simulink library "neuromorphic_blocks"  (R2022a)
settings: Solver=VariableStepAuto  StartTime=0.0  StopTime=10.0  RelTol=1e-3
libraries: $bdroot x47, simulink x7
(part 2 of 3)

== system neuromorphic_blocks/Neural Blocks ==
  Modulatory Synapse : Subsystem  mask(Modulatory Synapse){base_val=0, gsyn_pos_source=Internal, gsyn_pos=0, gsyn_neg_source=Internal, gsyn_neg=0, timescale=0.004, rel_timescale=1000, input=Events, dsyn_pos=0, dsyn_neg=0, msyn_pos=1, msyn_neg=1}
      mask prompts: base_val "Value"; gsyn_pos_source "Source"; gsyn_pos "Value"; gsyn_neg_source "Source"; gsyn_neg "Value"; timescale "Value"; rel_timescale "Value"; dsyn_pos "Value"; dsyn_neg "Value"; msyn_pos "Value"; msyn_neg "Value"
      mask init: same as neuromorphic_blocks/Auxiliary Blocks/Event-Triggered Relay
      mask TypeOptions gsyn_pos_source: Internal | External
      mask Callback gsyn_pos_source:
      | mask  = Simulink.Mask.get(gcb);
      |     switch mask.getParameter('gsyn_pos_source').Value
      |         case 'Internal'
      |             mask.getParameter('gsyn_pos').Enabled = 'on';
      |         case 'External'
      |             mask.getParameter('gsyn_pos').Enabled = 'off';
      |     end
      mask TypeOptions gsyn_neg_source: Internal | External
      mask Callback gsyn_neg_source:
      | mask  = Simulink.Mask.get(gcb);
      |     switch mask.getParameter('gsyn_neg_source').Value
      |         case 'Internal'
      |             mask.getParameter('gsyn_neg').Enabled = 'on';
      |         case 'External'
      |             mask.getParameter('gsyn_neg').Enabled = 'off';
      |     end
      mask TypeOptions input: Events | Voltage
      mask Callback input:
      | mask = Simulink.Mask.get(gcb);
      |     switch mask.getParameter('input').Value
      |         case 'Events'
      |             mask.getParameter('dsyn_pos').Enabled = 'off';
      |             mask.getParameter('dsyn_pos').Visible = 'off';
      |             mask.getDialogControl('dsyn_pos_text').Enabled = 'off';
      |             mask.getDialogControl('dsyn_pos_text').Visible = 'off';
      |             mask.getParameter('dsyn_neg').Enabled = 'off';
      |             mask.getParameter('dsyn_neg').Visible = 'off';
      |             mask.getDialogControl('dsyn_neg_text').Enabled = 'off';
      |             mask.getDialogControl('dsyn_neg_text').Visible = 'off';
      |             mask.getParameter('msyn_pos').Enabled = 'off';
      |             mask.getParameter('msyn_pos').Visible = 'off';
      |             mask.getDialogControl('msyn_pos_text').Enabled = 'off';
      |             mask.getDialogControl('msyn_pos_text').Visible = 'off';
      |             mask.getParameter('msyn_neg').Enabled = 'off';
      |             mask.getParameter('msyn_neg').Visible = 'off';
      |             mask.getDialogControl('msyn_neg_text').Enabled = 'off';
      |             mask.getDialogControl('msyn_neg_text').Visible = 'off';
      |         case 'Voltage'
      |             mask.getParameter('dsyn_pos').Enabled = 'on';
      |             mask.getParameter('dsyn_pos').Visible = 'on';
      |             mask.getDialogControl('dsyn_pos_text').Enabled = 'on';
      |             mask.getDialogControl('dsyn_pos_text').Visible = 'on';
      |             mask.getParameter('dsyn_neg').Enabled = 'on';
      |             mask.getParameter('dsyn_neg').Visible = 'on';
      |             mask.getDialogControl('dsyn_neg_text').Enabled = 'on';
      |             mask.getDialogControl('dsyn_neg_text').Visible = 'on';
      |             mask.getParameter('msyn_pos').Enabled = 'on';
      |             mask.getParameter('msyn_pos').Visible = 'on';
      |             mask.getDialogControl('msyn_pos_text').Enabled = 'on';
      |             mask.getDialogControl('msyn_pos_text').Visible = 'on';
      |             mask.getParameter('msyn_neg').Enabled = 'on';
      |             mask.getParameter('msyn_neg').Visible = 'on';
      |             mask.getDialogControl('msyn_neg_text').Enabled = 'on';
      |             mask.getDialogControl('msyn_neg_text').Visible = 'on';
      |     end
      mask DialogControl base_val_text Prompt: Start Parameter
      mask DialogControl gsyn_pos_text Prompt: Positive Event Conductance
      mask DialogControl gsyn_neg_text Prompt: Negative Event Conductance
      mask DialogControl timescale_text Prompt: Timescale
      mask DialogControl rel_timescale_text Prompt: Relative Timescale
      mask DialogControl input_text Prompt: Input Type
      mask DialogControl dsyn_pos_text Prompt: Positive Event Bias
      mask DialogControl dsyn_neg_text Prompt: Negative Event Bias
      mask DialogControl msyn_pos_text Prompt: Positive Event Gain
      mask DialogControl msyn_neg_text Prompt: Negative Event Gain
      mask Display:
      | image('icons/modulatory.jpg');
      | 
      | port_label('output', 1, 'p');
      | 
      | simBlockH = get_param(gcb, 'Handle');
      | portH = find_system(simBlockH, 'LookUnderMasks', 'on', 'FollowLinks', 'on', 'SearchDepth', 1, 'BlockType', 'Inport');
      | portNames = cellstr(get_param(portH, 'Name'));
      | portNum = cellstr(get_param(portH, 'Port'));
      | for i = 1:length(portNames)
      |     if ~isempty(portNames{i})
      |         num = str2num(['uint8(' portNum{i} ')']);
      |         port_label('input', num, portNames{i});
      |     end
      | end
  Neuron : Subsystem  mask(Neuron){gfm_source=Internal, gfm=0, gsp_source=Internal, gsp=0, gsm_source=Internal, gsm=0, gup_source=Internal, gup=0, gum_source=Internal, gum=0, dfm=0, dsp=0, dsm=0, dup=0, dum=0, mfm=1, msp=1, msm=1, mup=1, mum=1, timescale=0.004, rel_membrane=0.1, rel_fast=0.1, rel_slow=4, rel_ultraslow=200, Iapp_base=0, V0=0, tresh=0, output=Events}
      mask prompts: gfm_source "Source"; gfm "Value"; gsp_source "Source"; gsp "Value"; gsm_source "Source"; gsm "Value"; gup_source "Source"; gup "Value"; gum_source "Source"; gum "Value"; dfm "Value"; dsp "Value"; dsm "Value"; dup "Value"; dum "Value"; mfm "Value"; msp "Value"; msm "Value"; mup "Value"; mum "Value"; timescale "Value"; rel_membrane "Value"; rel_fast "Value"; rel_slow "Value"; rel_ultraslow "Value"; Iapp_base "Value"; V0 "Value"; tresh "Value"
      mask help:
      | Block simulating a simplified neuron model (L. Ribar and R. Sepulchre 2019).
      | The conductances can either be set or given as external inputs for neuromodulation.
      mask init:
      | mask  = Simulink.Mask.get(gcb);
      |     
      |     suffix_list = {'fm','sp','sm','up','um'};
      |     
      |     for suffix_cell = suffix_list
      |         suffix = suffix_cell{1};
      |         %block = find_system(gcb, 'LookUnderMasks', 'on', ...
      |         %                        'FollowLinks', 'on', 'Name', ['g' suffix]);
      |         %if isempty(block) 
      |             % Something is very wrong, recreate block
      |         %    add_block('built-in/Constant', [gcb '/g' suffix])
      |         %    h = get_param([gcb '/I' suffix],'LineHandles');
      |         %    if h.Inport(2) > 0
      |         %        delete_line(h.Inport(2)); 
      |         %    end 
      |         %    add_line(gcb,['g' suffix '/1'],['I' suffix '/2']);
      |         %end
      |     
      |         type = get_param([gcb '/g' suffix],'BlockType');
      |         switch mask.getParameter(['g' suffix '_source']).Value
      |             case 'Internal'
      |                 switch type
      |                     case 'Inport'
      |                         replace_block([gcb '/g' suffix], 'Inport', 'Constant', 'noprompt');
      |                         set_param([gcb '/g' suffix],'Value',['g' suffix]);
      |                 end
      |                 if strcmp('0', mask.getParameter(['g' suffix ]).Value)
      |                     set_param([gcb '/I' suffix],'Commented','on')
      |                     set_param([gcb '/g' suffix],'Commented','on')
      |                     set_param([gcb '/I' suffix '_sub'],'Commented','on')
      |                 else
      |                     set_param([gcb '/I' suffix],'Commented','off')
      |                     set_param([gcb '/g' suffix],'Commented','off')
      |                     set_param([gcb '/I' suffix '_sub'],'Commented','off')
      |                 end
      |             case 'External'
      |                 switch type
      |                     case 'Constant'
      |                         replace_block([gcb '/g' suffix], 'Constant', 'Inport', 'noprompt');
      |                 end
      |                 set_param([gcb '/I' suffix],'Commented','off')
      |                 set_param([gcb '/g' suffix],'Commented','off')
      |                 set_param([gcb '/I' suffix '_sub'],'Commented','off')
      |         end
      |     end
      | 
      |     type_V = get_param([gcb '/V'],'BlockType');
      |     type_Ev = get_param([gcb '/Ev'],'BlockType');
      |     switch mask.getParameter('output').Value
      |         case 'Events'
      |             switch type_V
      |                 case 'Outport'
      |                     replace_block([gcb '/V'], 'Outport', 'Terminator', 'noprompt')
      |             end
      |             switch type_Ev
      |                 case 'Terminator'
      |                     replace_block([gcb '/Ev'], 'Terminator', 'Outport', 'noprompt')
      |             end
      |             set_param([gcb '/V_to_Ev'],'Commented','off')
      |         case 'Voltage'
      |             switch type_V
      |                 case 'Terminator'
      |                     replace_block([gcb '/V'], 'Terminator', 'Outport', 'noprompt')
      |             end
      |             switch type_Ev
      |                 case 'Outport'
      |                     replace_block([gcb '/Ev'], 'Outport', 'Terminator', 'noprompt')
      |             end
      |             set_param([gcb '/V_to_Ev'],'Commented','on')
      |         case 'Both'
      |             switch type_Ev
      |                 case 'Terminator'
      |                     switch type_V
      |                         case 'Outport'
      |                             replace_block([gcb '/V'], 'Outport', 'Terminator', 'noprompt')
      |                             type_V = 'Terminator';
      |                     end
      |                     replace_block([gcb '/Ev'], 'Terminator', 'Outport', 'noprompt')
      |             end
      |             switch type_V
      |                 case 'Terminator'
      |                     replace_block([gcb '/V'], 'Terminator', 'Outport', 'noprompt')
      |             end
      |             set_param([gcb '/V_to_Ev'],'Commented','off')
      |     end
      mask TypeOptions gfm_source: Internal | External
      mask Callback gfm_source:
      | source_name = 'gfm_source';
      |     tgt_name = 'gfm';
      |     mask  = Simulink.Mask.get(gcb);
      |     switch mask.getParameter(source_name).Value
      |         case 'Internal'
      |             mask.getParameter(tgt_name).Enabled = 'on';
      |         case 'External'
      |             mask.getParameter(tgt_name).Enabled = 'off';
      |     end
      mask TypeOptions gsp_source: Internal | External
      mask Callback gsp_source:
      | source_name = 'gsp_source';
      |     tgt_name = 'gsp';
      |     mask  = Simulink.Mask.get(gcb);
      |     switch mask.getParameter(source_name).Value
      |         case 'Internal'
      |             mask.getParameter(tgt_name).Enabled = 'on';
      |         case 'External'
      |             mask.getParameter(tgt_name).Enabled = 'off';
      |     end
      mask TypeOptions gsm_source: Internal | External
      mask Callback gsm_source:
      | source_name = 'gsm_source';
      |     tgt_name = 'gsm';
      |     mask  = Simulink.Mask.get(gcb);
      |     switch mask.getParameter(source_name).Value
      |         case 'Internal'
      |             mask.getParameter(tgt_name).Enabled = 'on';
      |         case 'External'
      |             mask.getParameter(tgt_name).Enabled = 'off';
      |     end
      mask TypeOptions gup_source: Internal | External
      mask Callback gup_source:
      | source_name = 'gup_source';
      |     tgt_name = 'gup';
      |     mask  = Simulink.Mask.get(gcb);
      |     switch mask.getParameter(source_name).Value
      |         case 'Internal'
      |             mask.getParameter(tgt_name).Enabled = 'on';
      |         case 'External'
      |             mask.getParameter(tgt_name).Enabled = 'off';
      |     end
      mask TypeOptions gum_source: Internal | External
      mask Callback gum_source:
      | source_name = 'gum_source';
      |     tgt_name = 'gum';
      |     mask  = Simulink.Mask.get(gcb);
      |     switch mask.getParameter(source_name).Value
      |         case 'Internal'
      |             mask.getParameter(tgt_name).Enabled = 'on';
      |         case 'External'
      |             mask.getParameter(tgt_name).Enabled = 'off';
      |     end
      mask TypeOptions output: Events | Voltage | Both
      mask Callback output:
      | source_name = 'output';
      |     tgt_name = 'tresh';
      |     mask  = Simulink.Mask.get(gcb);
      |     switch mask.getParameter(source_name).Value
      |         case 'Voltage'
      |             mask.getParameter(tgt_name).Enabled = 'off';
      |         otherwise
      |             mask.getParameter(tgt_name).Enabled = 'on';
      |     end
      mask DialogControl ConductancesContainer Prompt: Conductances
      mask DialogControl gfm_text Prompt: Fast Negative Conductance (gfm)
      mask DialogControl gsp_text Prompt: Slow Positive Conductance (gsp)
      mask DialogControl gsm_text Prompt: Slow Negative Conductance (gsm)
      mask DialogControl gup_text Prompt: Ultra-Slow Positive Conductance (gup)
      mask DialogControl gum_text Prompt: Ultra-Slow Negative Conductance (gum)
      mask DialogControl BiasesContainer Prompt: Biases
      mask DialogControl dfm_text Prompt: Fast Negative Bias (dfm)
      mask DialogControl dsp_text Prompt: Slow Positive Bias (dsp)
      mask DialogControl dsm_text Prompt: Slow Negative Bias (dsm)
      mask DialogControl dup_text Prompt: Ultra-Slow Positive Bias (gup)
      mask DialogControl dum_text Prompt: Ultra-Slow Negative Bias (gum)
      mask DialogControl SlopesContainer Prompt: Slopes
      mask DialogControl mfm_text Prompt: Fast Negative Slope (mfm)
      mask DialogControl msp_text Prompt: Slow Positive Slope (msp)
      mask DialogControl msm_text Prompt: Slow Negative Slope (msm)
      mask DialogControl mup_text Prompt: Ultra-Slow Positive Slope (mup)
      mask DialogControl mum_text Prompt: Ultra-Slow Negative Slope (mum)
      mask DialogControl TimescalesContainer Prompt: Timescales
      mask DialogControl timescale_text Prompt: Timescale
      mask DialogControl memb_text Prompt: Relative Membrane Timescale
      mask DialogControl fast_text Prompt: Relative Fast Timescale
      mask DialogControl slow_text Prompt: Relative Slow Timescale
      mask DialogControl ultraslow_text Prompt: Relative Ultra-Slow Timescale
      mask DialogControl OtherContainer Prompt: Other
      mask DialogControl Iapp_text Prompt: Base Applied Current
      mask DialogControl V0_text Prompt: Base Voltage
      mask DialogControl tresh_text Prompt: Event Threshold
      mask DialogControl output_text Prompt: Output
      mask Display:
      | pos = get_param(gcb, 'Position');
      | width = pos(3) - pos(1);
      | height = pos(4) - pos(2);
      | 
      | image('icons/neuron.jpg');
      | 
      | simBlockH = get_param(gcb, 'Handle');
      | 
      | 
      | portH = find_system(simBlockH, 'LookUnderMasks', 'on', 'FollowLinks', 'on', 'SearchDepth', 1, 'BlockType', 'Inport');
      | portNames = cellstr(get_param(portH, 'Name'));
      | portNum = cellstr(get_param(portH, 'Port'));
      | for i = 1:length(portNames)
      |     if ~isempty(portNames{i})
      |         num = str2num(['uint8(' portNum{i} ')']);
      |         port_label('input', num, portNames{i});
      |     end
      | end
      | 
      | portH = find_system(simBlockH, 'LookUnderMasks', 'on', 'FollowLinks', 'on', 'SearchDepth', 1, 'BlockType', 'Outport');
      | portNames = cellstr(get_param(portH, 'Name'));
      | portNum = cellstr(get_param(portH, 'Port'));
      | for i = 1:length(portNames)
      |     if ~isempty(portNames{i})
      |         num = str2num(['uint8(' portNum{i} ')']);
      |         port_label('output', num, portNames{i});
      |     end
      | end
  Synapse with Depression : Subsystem  mask(Synapse with Depression){gsyn_source=Internal, gsyn=0, dsyn=0, msyn=1, dsyn_dep=0, msyn_dep=1, timescale=0.004, rel_facilitation=0, rel_depression=100, input=Events, gsyn_in=0, dsyn_in=0, msyn_in=1}
      mask prompts: gsyn_source "Source"; gsyn "Value"; dsyn "Value"; msyn "Value"; dsyn_dep "Value"; msyn_dep "Value"; timescale "Value"; rel_facilitation "Value"; rel_depression "Value"; gsyn_in "Value"; dsyn_in "Value"; msyn_in "Value"
      mask help: Synapse that lets through the first spikes
      mask init:
      | mask  = Simulink.Mask.get(gcb);
      |     %block = find_system(gcb, 'LookUnderMasks', 'on', ...
      |     %                    'FollowLinks', 'on', 'Name', 'gsyn');
      |     %if isempty(block) 
      |         % Something is very wrong, recreate block
      |     %    add_block('built-in/Constant', [gcb '/gsyn'])
      |     %    h = get_param([gcb '/Sigmoid'],'LineHandles');
      |     %    if h.Inport(2) > 0
      |     %        delete_line(h.Inport(2)); 
      |     %    end 
      |     %    add_line(gcb,'gsyn/1','Sigmoid/2');
      |     %    h = get_param([gcb '/Out Depression Sigmoid'],'LineHandles');
      |     %    if h.Inport(2) > 0
      |     %        delete_line(h.Inport(2)); 
      |     %    end 
      |     %    add_line(gcb,'gsyn/1','Out Depression Sigmoid/2');
      |     %end
      | 
      |     switch mask.getParameter('input').Value
      |         case 'Events'
      |             set_param([gcb '/VSNK' ],'LabelModeActiveChoice', 'Events');
      |             set_param([gcb '/VSRC' ],'LabelModeActiveChoice', 'Events');
      |             %mask.getPortConstraint('in_main_type').Rule.DataType = {'boolean'};
      |             try
      |                 set_param([gcb '/V'], 'Name', 'Ev');
      |             catch E
      |             end
      |         case 'Voltage'
      |             set_param([gcb '/VSNK' ],'LabelModeActiveChoice', 'Voltage');
      |             set_param([gcb '/VSRC' ],'LabelModeActiveChoice', 'Voltage');
      |             %mask.getPortConstraint('in_main_type').Rule.DataType = {'double'; 'single'; 'int8'; 'uint8'; 'int16'; 'uint16'; 'int32'; 'uint32'};
      |             try
      |                 set_param([gcb '/Ev'], 'Name', 'V');
      |             catch E
      |             end
      |     end
      | 
      |     switch mask.getParameter('gsyn_source').Value
      |         case 'Internal'
      |             replace_block([gcb '/gsyn'], 'Inport', 'Constant', 'noprompt');
      |             set_param([gcb '/gsyn'],'Value','gsyn');
      |         case 'External'
      |             replace_block([gcb '/gsyn'], 'Constant', 'Inport', 'noprompt');
      |     end
      mask TypeOptions gsyn_source: Internal | External
      mask Callback gsyn_source:
      | mask  = Simulink.Mask.get(gcb);
      |     switch mask.getParameter('gsyn_source').Value
      |         case 'Internal'
      |             mask.getParameter('gsyn').Enabled = 'on';
      |         case 'External'
      |             mask.getParameter('gsyn').Enabled = 'off';
      |     end
      mask TypeOptions input: Events | Voltage
      mask Callback input:
      | mask = Simulink.Mask.get(gcb);
      |     switch mask.getParameter('input').Value
      |         case 'Events'
      |             mask.getParameter('gsyn_in').Enabled = 'off';
      |             mask.getParameter('gsyn_in').Visible = 'off';
      |             mask.getDialogControl('gsyn_in_text').Enabled = 'off';
      |             mask.getDialogControl('gsyn_in_text').Visible = 'off';
      |             mask.getParameter('dsyn_in').Enabled = 'off';
      |             mask.getParameter('dsyn_in').Visible = 'off';
      |             mask.getDialogControl('dsyn_in_text').Enabled = 'off';
      |             mask.getDialogControl('dsyn_in_text').Visible = 'off';
      |             mask.getParameter('msyn_in').Enabled = 'off';
      |             mask.getParameter('msyn_in').Visible = 'off';
      |             mask.getDialogControl('msyn_in_text').Enabled = 'off';
      |             mask.getDialogControl('msyn_in_text').Visible = 'off';
      |         case 'Voltage'
      |             mask.getParameter('gsyn_in').Enabled = 'on';
      |             mask.getParameter('gsyn_in').Visible = 'on';
      |             mask.getDialogControl('gsyn_in_text').Enabled = 'on';
      |             mask.getDialogControl('gsyn_in_text').Visible = 'on';
      |             mask.getParameter('dsyn_in').Enabled = 'on';
      |             mask.getParameter('dsyn_in').Visible = 'on';
      |             mask.getDialogControl('dsyn_in_text').Enabled = 'on';
      |             mask.getDialogControl('dsyn_in_text').Visible = 'on';
      |             mask.getParameter('msyn_in').Enabled = 'on';
      |             mask.getParameter('msyn_in').Visible = 'on';
      |             mask.getDialogControl('msyn_in_text').Enabled = 'on';
      |             mask.getDialogControl('msyn_in_text').Visible = 'on';
      |     end
      mask DialogControl gsyn_text Prompt: Conductance (gsyn)
      mask DialogControl dsyn_text Prompt: Bias (dsyn)
      mask DialogControl msyn_text Prompt: Slope (msyn)
      mask DialogControl dsyn_dep_text Prompt: Depression Bias (dsyn_dep)
      mask DialogControl msyn_dep_text Prompt: Depression Slope (msyn_dep)
      mask DialogControl timescale_text Prompt: Timescale
      mask DialogControl rel_facilitation_text Prompt: Facilitation Timescale
      mask DialogControl rel_depression_text Prompt: Depression Timescale
      mask DialogControl input_text Prompt: Input Type
      mask DialogControl gsyn_in_text Prompt: Input Conductance (gsyn_in)
      mask DialogControl dsyn_in_text Prompt: Inout Bias (dsyn_in)
      mask DialogControl msyn_in_text Prompt: Input Slope (msyn_in)
      mask Display:
      | mask  = Simulink.Mask.get(gcb);
      | [gsyn, gsyn_converted] = str2num(mask.getParameter('gsyn').Value);
      | [msyn, msyn_converted] = str2num(mask.getParameter('msyn').Value);
      | 
      | if strcmp(mask.getParameter('gsyn_source').Value,'Internal') ...
      |    && gsyn_converted && msyn_converted && gsyn*msyn < 0
      |     image('icons/depressing_inhib_syn.jpg');
      | else
      |     image('icons/depressing_excit_syn.jpg');
      | end
      | 
      | port_label('output', 1, 'Isyn');
      | 
      | simBlockH = get_param(gcb, 'Handle');
      | portH = find_system(simBlockH, 'LookUnderMasks', 'on', 'FollowLinks', 'on', 'SearchDepth', 1, 'BlockType', 'Inport');
      | portNames = cellstr(get_param(portH, 'Name'));
      | portNum = cellstr(get_param(portH, 'Port'));
      | for i = 1:length(portNames)
      |     if ~isempty(portNames{i})
      |         num = str2num(['uint8(' portNum{i} ')']);
      |         port_label('input', num, portNames{i});
      |     end
      | end
  Synapse with Facilitation : Subsystem  mask(Synapse with Facilitation){gsyn_source=Internal, gsyn=0, dsyn=0, msyn=1, timescale=0.004, rel_timescale=10, input=Events, gsyn_in=0, dsyn_in=0, msyn_in=1}
      mask prompts: gsyn_source "Source"; gsyn "Value"; dsyn "Value"; msyn "Value"; timescale "Value"; rel_timescale "Value"; gsyn_in "Value"; dsyn_in "Value"; msyn_in "Value"
      mask help: Synapse that transmit well long packets of spikes
      mask init:
      | mask  = Simulink.Mask.get(gcb);
      |     %block = find_system(gcb, 'LookUnderMasks', 'on', ...
      |     %                    'FollowLinks', 'on', 'Name', 'gsyn');
      |     %if isempty(block) 
      |     %    % Something is very wrong, recreate block
      |     %    add_block('built-in/Constant', [gcb '/gsyn'])
      |     %    h = get_param([gcb '/sigmoid'],'LineHandles');
      |     %    if h.Inport(2) > 0
      |     %        delete_line(h.Inport(2)); 
      |     %    end 
      |     %    add_line(gcb,'gsyn/1','sigmoid/2');
      |     %end
      | 
      |     %result = find_system([gcb], 'type', 'Block')
      |     %disp(result)
      |     %disp(gcb)
      | 
      |     switch mask.getParameter('input').Value
      |         case 'Events'
      |             set_param([gcb '/VSNK' ],'LabelModeActiveChoice', 'Events');
      |             set_param([gcb '/VSRC' ],'LabelModeActiveChoice', 'Events');
      |             %mask.getPortConstraint('in_main_type').Rule.DataType = {'boolean'};
      |             try
      |                 set_param([gcb '/V'], 'Name', 'Ev');
      |             catch E
      |             end
      |         case 'Voltage'
      |             set_param([gcb '/VSNK' ],'LabelModeActiveChoice', 'Voltage');
      |             set_param([gcb '/VSRC' ],'LabelModeActiveChoice', 'Voltage');
      |             %mask.getPortConstraint('in_main_type').Rule.DataType = {'double'; 'single'; 'int8'; 'uint8'; 'int16'; 'uint16'; 'int32'; 'uint32'};
      |             try
      |                 set_param([gcb '/Ev'], 'Name', 'V');
      |             catch E
      |             end
      |     end
      | 
      |     switch mask.getParameter('gsyn_source').Value
      |         case 'Internal'
      |             replace_block([gcb '/gsyn'], 'Inport', 'Constant', 'noprompt');
      |             set_param([gcb '/gsyn'],'Value','gsyn');
      |         case 'External'
      |             replace_block([gcb '/gsyn'], 'Constant', 'Inport', 'noprompt');
      |     end
      mask TypeOptions gsyn_source: Internal | External
      mask Callback gsyn_source:
      | mask = Simulink.Mask.get(gcb);
      |     switch mask.getParameter('gsyn_source').Value
      |         case 'Internal'
      |             mask.getParameter('gsyn').Enabled = 'on';
      |         case 'External'
      |             mask.getParameter('gsyn').Enabled = 'off';
      |     end
      mask TypeOptions input: Events | Voltage
      mask Callback input:
      | mask = Simulink.Mask.get(gcb);
      |     switch mask.getParameter('input').Value
      |         case 'Events'
      |             mask.getParameter('gsyn_in').Enabled = 'off';
      |             mask.getParameter('gsyn_in').Visible = 'off';
      |             mask.getDialogControl('gsyn_in_text').Enabled = 'off';
      |             mask.getDialogControl('gsyn_in_text').Visible = 'off';
      |             mask.getParameter('dsyn_in').Enabled = 'off';
      |             mask.getParameter('dsyn_in').Visible = 'off';
      |             mask.getDialogControl('dsyn_in_text').Enabled = 'off';
      |             mask.getDialogControl('dsyn_in_text').Visible = 'off';
      |             mask.getParameter('msyn_in').Enabled = 'off';
      |             mask.getParameter('msyn_in').Visible = 'off';
      |             mask.getDialogControl('msyn_in_text').Enabled = 'off';
      |             mask.getDialogControl('msyn_in_text').Visible = 'off';
      |         case 'Voltage'
      |             mask.getParameter('gsyn_in').Enabled = 'on';
      |             mask.getParameter('gsyn_in').Visible = 'on';
      |             mask.getDialogControl('gsyn_in_text').Enabled = 'on';
      |             mask.getDialogControl('gsyn_in_text').Visible = 'on';
      |             mask.getParameter('dsyn_in').Enabled = 'on';
      |             mask.getParameter('dsyn_in').Visible = 'on';
      |             mask.getDialogControl('dsyn_in_text').Enabled = 'on';
      |             mask.getDialogControl('dsyn_in_text').Visible = 'on';
      |             mask.getParameter('msyn_in').Enabled = 'on';
      |             mask.getParameter('msyn_in').Visible = 'on';
      |             mask.getDialogControl('msyn_in_text').Enabled = 'on';
      |             mask.getDialogControl('msyn_in_text').Visible = 'on';
      |     end
      mask DialogControl gsyn_text Prompt: Conductance (gsyn)
      mask DialogControl dsyn_text Prompt: Bias (dsyn)
      mask DialogControl msyn_text Prompt: Slope (msyn)
      mask DialogControl timescale_text Prompt: Timescale
      mask DialogControl rel_text Prompt: Relative Timescale
      mask DialogControl input_text Prompt: Input Type
      mask DialogControl gsyn_in_text Prompt: Input Conductance (gsyn_in)
      mask DialogControl dsyn_in_text Prompt: Input Bias (dsyn_in)
      mask DialogControl msyn_in_text Prompt: Input Slope (msyn_in)
      mask Display:
      | mask  = Simulink.Mask.get(gcb);
      | [gsyn, gsyn_converted] = str2num(mask.getParameter('gsyn').Value);
      | [msyn, msyn_converted] = str2num(mask.getParameter('msyn').Value);
      | 
      | if strcmp(mask.getParameter('gsyn_source').Value,'Internal') ...
      |    && gsyn_converted && msyn_converted && gsyn*msyn < 0
      |     image('icons/facilitating_inhib_syn.jpg');
      | else
      |     image('icons/facilitating_excit_syn.jpg');
      | end
      | 
      | 
      | port_label('output', 1, 'Isyn');
      | 
      | simBlockH = get_param(gcb, 'Handle');
      | portH = find_system(simBlockH, 'LookUnderMasks', 'on', 'FollowLinks', 'on', 'SearchDepth', 1, 'BlockType', 'Inport');
      | portNames = cellstr(get_param(portH, 'Name'));
      | portNum = cellstr(get_param(portH, 'Port'));
      | for i = 1:length(portNames)
      |     if ~isempty(portNames{i})
      |         num = str2num(['uint8(' portNum{i} ')']);
      |         port_label('input', num, portNames{i});
      |     end
      | end

== system neuromorphic_blocks/Quick Insert ==
  Neural Blocks : Subsystem
      mask Display: disp("Neural Blocks")

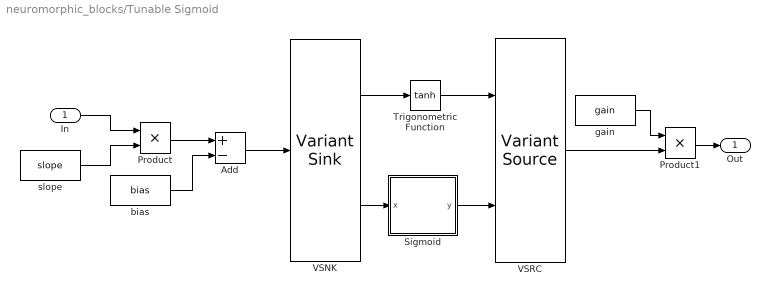
== system neuromorphic_blocks/Tunable Sigmoid ==
  In : Inport
  Add : Sum  Inputs=+-
  Product : Product
  Product1 : Product
  Sigmoid : Subsystem
  Trigonometric Function : Trigonometry  Operator=tanh
  VSNK : VariantSink  VariantControlMode=label  LabelModeActiveChoice=Sigmoid  ShowConditionOnBlock=on
  VSRC : VariantSource  VariantControlMode=label  LabelModeActiveChoice=Sigmoid  ShowConditionOnBlock=on
  bias : Constant  Value=bias
  gain : Constant  Value=gain
  slope : Constant  Value=slope
  Out : Outport
  wires:
  VSNK/1 -> Trigonometric Function/1
  slope/1 -> Product/2
  In/1 -> Product/1
  Add/1 -> VSNK/1
  Product/1 -> Add/1
  bias/1 -> Add/2
  VSRC/1 -> Product1/2
  Product1/1 -> Out/1
  gain/1 -> Product1/1
  VSNK/2 -> Sigmoid/1(x)
  Sigmoid/1(y) -> VSRC/2
  Trigonometric Function/1 -> VSRC/1

== system neuromorphic_blocks/Auxiliary Blocks/Directional Threshold Detector ==
  s : Inport
  In Sigmoid : $bdroot/Tunable Sigmoid  nonlinearity_type=Sigmoid  gain_source=Internal  gain=gain_in  bias=bias_in  slope=slope_in
  Out Sigmoid : $bdroot/Tunable Sigmoid  nonlinearity_type=Sigmoid  gain_source=Internal  gain=gain_out  bias=bias_out  slope=slope_out
  Rebound Neuron : $bdroot/Neural Blocks/Neuron  gfm_source=Internal  gfm=gfm  gsp_source=Internal  gsp=gsp  gsm_source=Internal  gsm=0  gup_source=Internal  gup=gup  gum_source=Internal  gum=0  dfm=dfm  dsp=dsp  dsm=0  dup=dup  dum=0  mfm=mfm  msp=msp  msm=1  mup=mup  mum=1  timescale=timescale  rel_membrane=rel_membrane  rel_fast=rel_fast  rel_slow=rel_slow  rel_ultraslow=1  Iapp_base=Iapp_base  V0=V0  tresh=tresh  output=Both
  V : Terminator
  Ev : Outport
  wires:
  s/1 -> In Sigmoid/1
  In Sigmoid/1 -> Rebound Neuron/1
  Rebound Neuron/1 -> Ev/1
  Rebound Neuron/2 -> Out Sigmoid/1
  Out Sigmoid/1 -> V/1

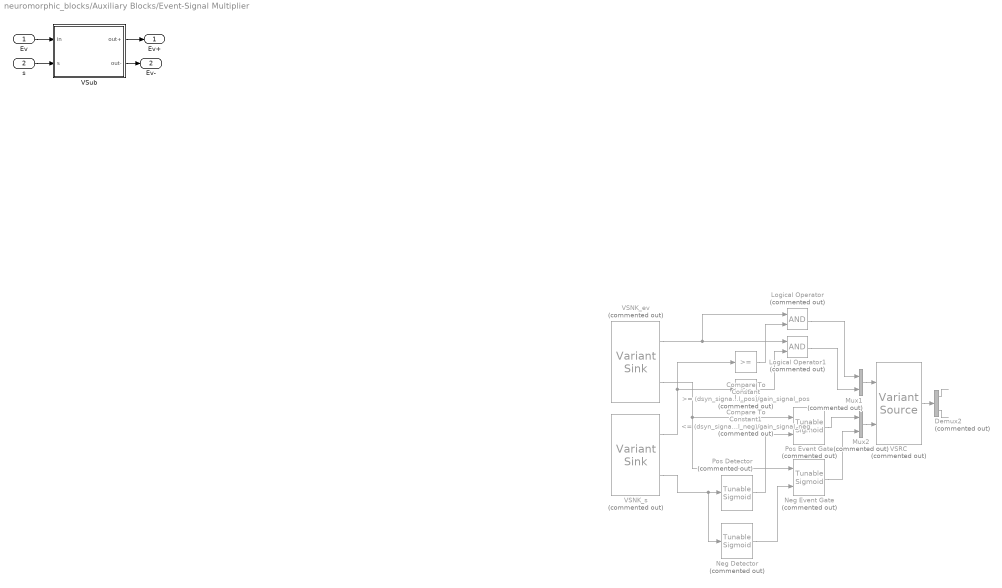
== system neuromorphic_blocks/Auxiliary Blocks/Event-Signal Multiplier ==
  Ev : Inport
  s : Inport  Port=2
  Compare To Constant : simulink/Logic and Bit Operations/Compare To Constant  Commented=on  relop=>=  const=(dsyn_signal_pos)/gain_signal_pos  OutDataTypeStr=boolean
  Compare To Constant1 : simulink/Logic and Bit Operations/Compare To Constant  Commented=on  relop=<=  const=(dsyn_signal_neg)/gain_signal_neg  OutDataTypeStr=boolean
  Demux2 : Demux  Commented=on  Outputs=2
  Logical Operator : Logic  Commented=on  AllPortsSameDT=off  OutDataTypeStr=boolean
  Logical Operator1 : Logic  Commented=on  AllPortsSameDT=off  OutDataTypeStr=boolean
  Mux1 : Mux  Commented=on  Inputs=2
  Mux2 : Mux  Commented=on  Inputs=2
  Neg Detector : $bdroot/Tunable Sigmoid  Commented=on  nonlinearity_type=Sigmoid  gain_source=Internal  gain=gsyn_neg  bias=-dsyn_signal_neg  slope=-gain_signal_neg
  Neg Event Gate : $bdroot/Tunable Sigmoid  Commented=on  nonlinearity_type=Sigmoid  gain_source=External  gain=0  bias=dsyn_event_neg  slope=gain_event_neg
  Pos Detector : $bdroot/Tunable Sigmoid  Commented=on  nonlinearity_type=Sigmoid  gain_source=Internal  gain=gsyn_pos  bias=dsyn_signal_pos  slope=gain_signal_pos
  Pos Event Gate : $bdroot/Tunable Sigmoid  Commented=on  nonlinearity_type=Sigmoid  gain_source=External  gain=0  bias=dsyn_event_pos  slope=gain_event_pos
  VSNK_ev : VariantSink  Commented=on  VariantControlMode=label  LabelModeActiveChoice=Events  ShowConditionOnBlock=on
  VSNK_s : VariantSink  Commented=on  VariantControlMode=label  LabelModeActiveChoice=Events  ShowConditionOnBlock=on
  VSRC : VariantSource  Commented=on  VariantControlMode=label  LabelModeActiveChoice=Events  ShowConditionOnBlock=on
  VSub : Subsystem  Variant=on  VariantControlMode=label  LabelModeActiveChoice=Events
  Ev+ : Outport
  Ev- : Outport  Port=2
  wires:
  Ev/1 -> VSub/1(in)
  s/1 -> VSub/2(s)
  Logical Operator1/1 -> Mux1/2
  Demux2/2 -> ?
  Mux2/1 -> VSRC/2
  VSNK_ev/2 -> Neg Event Gate/1, Pos Event Gate/1
  VSNK_s/1 -> Compare To Constant/1, Compare To Constant1/1
  Logical Operator/1 -> Mux1/1
  Demux2/1 -> ?
  Neg Detector/1 -> Neg Event Gate/2
  VSRC/1 -> Demux2/1
  VSNK_ev/1 -> Logical Operator1/1, Logical Operator/1
  Neg Event Gate/1 -> Mux2/2
  Mux1/1 -> VSRC/1
  Pos Detector/1 -> Pos Event Gate/2
  VSNK_s/2 -> Neg Detector/1, Pos Detector/1
  Compare To Constant/1 -> Logical Operator/2
  Compare To Constant1/1 -> Logical Operator1/2
  Pos Event Gate/1 -> Mux2/1
  VSub/2(out-) -> Ev-/1
  VSub/1(out+) -> Ev+/1

== system neuromorphic_blocks/Auxiliary Blocks/Event-Signal Selector ==
  Ev+ : Inport
  Ev- : Inport  Port=2
  s : Inport  Port=3
  VSub : Subsystem  Variant=on  VariantControlMode=label  LabelModeActiveChoice=Events
  Ev : Outport
  wires:
  Ev+/1 -> VSub/1(in+)
  Ev-/1 -> VSub/2(in-)
  VSub/1(out) -> Ev/1
  s/1 -> VSub/3(s)

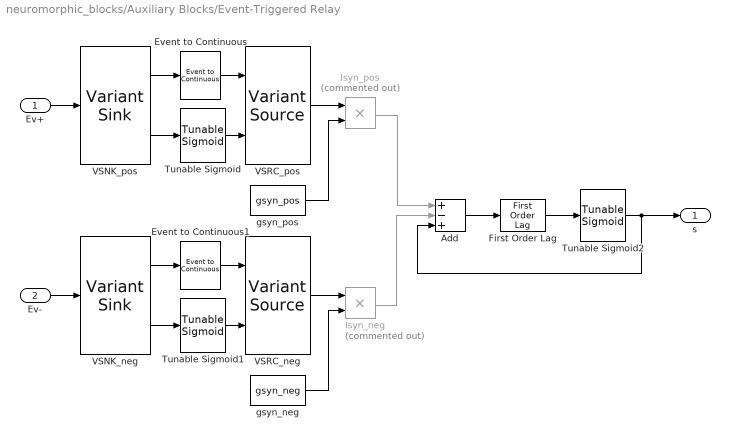
== system neuromorphic_blocks/Auxiliary Blocks/Event-Triggered Relay ==
  Ev+ : Inport
  Ev- : Inport  Port=2
  Add : Sum  Inputs=+-+
  Event to Continuous : $bdroot/Events Transmission Blocks/Event to Continuous  gain=1
  Event to Continuous1 : $bdroot/Events Transmission Blocks/Event to Continuous  gain=1
  First Order Lag : $bdroot/First Order Lag  gain=1  timescale=timescale  rel_timescale=rel_timescale
  Isyn_neg : Product  Commented=on
  Isyn_pos : Product  Commented=on
  Tunable Sigmoid : $bdroot/Tunable Sigmoid  nonlinearity_type=Sigmoid  gain_source=Internal  gain=1  bias=dsyn_pos  slope=msyn_pos
  Tunable Sigmoid1 : $bdroot/Tunable Sigmoid  nonlinearity_type=Sigmoid  gain_source=Internal  gain=1  bias=dsyn_neg  slope=msyn_neg
  Tunable Sigmoid2 : $bdroot/Tunable Sigmoid  nonlinearity_type=Sigmoid  gain_source=Internal  gain=gsyn_out  bias=dsyn_out  slope=msyn_out
  VSNK_neg : VariantSink  VariantControlMode=label  LabelModeActiveChoice=Events  ShowConditionOnBlock=on
  VSNK_pos : VariantSink  VariantControlMode=label  LabelModeActiveChoice=Events  ShowConditionOnBlock=on
  VSRC_neg : VariantSource  VariantControlMode=label  LabelModeActiveChoice=Events  ShowConditionOnBlock=on
  VSRC_pos : VariantSource  VariantControlMode=label  LabelModeActiveChoice=Events  ShowConditionOnBlock=on
  gsyn_neg : Constant  Value=gsyn_neg
  gsyn_pos : Constant  Value=gsyn_pos
  s : Outport
  wires:
  Ev+/1 -> VSNK_pos/1
  Isyn_pos/1 -> Add/1
  Isyn_neg/1 -> Add/2
  VSNK_pos/1 -> Event to Continuous/1
  Event to Continuous/1 -> VSRC_pos/1
  Tunable Sigmoid/1 -> VSRC_pos/2
  VSNK_pos/2 -> Tunable Sigmoid/1
  VSRC_pos/1 -> Isyn_pos/1
  gsyn_pos/1 -> Isyn_pos/2
  VSRC_neg/1 -> Isyn_neg/1
  gsyn_neg/1 -> Isyn_neg/2
  Event to Continuous1/1 -> VSRC_neg/1
  VSNK_neg/2 -> Tunable Sigmoid1/1
  VSNK_neg/1 -> Event to Continuous1/1
  Tunable Sigmoid1/1 -> VSRC_neg/2
  Ev-/1 -> VSNK_neg/1
  Add/1 -> First Order Lag/1
  Tunable Sigmoid2/1 -> s/1, Add/3
  First Order Lag/1 -> Tunable Sigmoid2/1

== system neuromorphic_blocks/Auxiliary Blocks/Noise on Signal ==
  In : Inport
  Add : Sum
  Noise : simulink/Sources/Band-Limited White Noise  Cov=noise_pwr  Ts=timescale*rel_timescale  seed=seed_mem
  Out : Outport
  wires:
  In/1 -> Add/2
  Add/1 -> Out/1
  Noise/1 -> Add/1

== system neuromorphic_blocks/Events Transmission Blocks/Continuous to Event ==
  In : Inport
  Constant2 : Constant  Value=thresh
  Relational Operator : RelationalOperator  OutDataTypeStr=boolean  RndMeth=Simplest  InputSameDT=off
  Out : Outport  OutDataTypeStr=boolean
  wires:
  Constant2/1 -> Relational Operator/2
  In/1 -> Relational Operator/1
  Relational Operator/1 -> Out/1

== system neuromorphic_blocks/Events Transmission Blocks/Event Loss ==
  In : Inport
  Constant4 : Constant  Value=0  OutDataTypeStr=Inherit: Inherit via back propagation
  Generate Random Number on Positive : Subsystem  TreatAsAtomicUnit=on
  Pipe Signal : Switch  Threshold=loss_prob  SaturateOnIntegerOverflow=off  InputSameDT=off
  Out : Outport
  wires:
  Generate Random Number on Positive/1(Out1) -> Pipe Signal/2
  In/1 -> Pipe Signal/1, Generate Random Number on Positive/Trigger
  Constant4/1 -> Pipe Signal/3
  Pipe Signal/1 -> Out/1

== system neuromorphic_blocks/Events Transmission Blocks/Event to Continuous ==
  In : Inport  OutDataTypeStr=boolean
  Gain : Gain  Gain=gain  OutDataTypeStr=double
  Out : Outport  OutDataTypeStr=double
  wires:
  In/1 -> Gain/1
  Gain/1 -> Out/1

== system neuromorphic_blocks/Events Transmission Blocks/Event to Fixed Width Pulse ==
  In : Inport  OutDataTypeStr=boolean
  Add : Sum  Inputs=+-
  Clock : Clock
  Constant : Constant  Value=pulse_width
  Relational Operator : RelationalOperator  Operator=>  OutDataTypeStr=boolean  RndMeth=Simplest  InputSameDT=off
  Triggered Subsystem : Subsystem  TreatAsAtomicUnit=on
  Out : Outport
  wires:
  Constant/1 -> Add/2
  Triggered Subsystem/1(Out1) -> Relational Operator/1
  Add/1 -> Relational Operator/2
  Clock/1 -> Add/1, Triggered Subsystem/1(In1)
  Relational Operator/1 -> Out/1
  In/1 -> Triggered Subsystem/Trigger

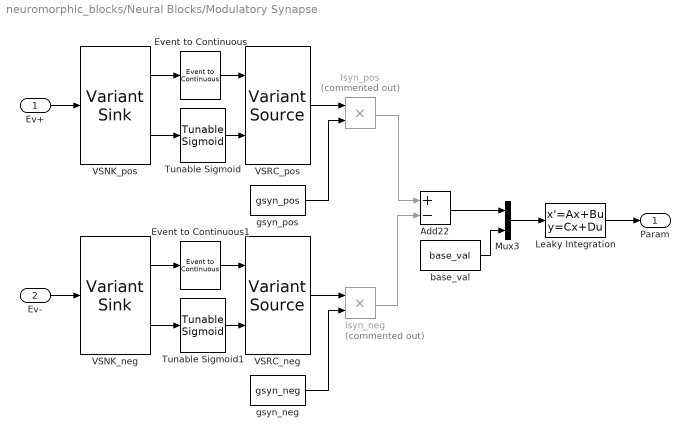
== system neuromorphic_blocks/Neural Blocks/Modulatory Synapse ==
  Ev+ : Inport
  Ev- : Inport  Port=2
  Add22 : Sum  Inputs=+-
  Event to Continuous : $bdroot/Events Transmission Blocks/Event to Continuous  gain=1
  Event to Continuous1 : $bdroot/Events Transmission Blocks/Event to Continuous  gain=1
  Isyn_neg : Product  Commented=on
  Isyn_pos : Product  Commented=on
  Leaky Integration : StateSpace  A=-1/(timescale*rel_timescale)  B=[1 1/(timescale*rel_timescale)]  D=[0 0]  InitialCondition=base_val  ParameterTunability=Unconstrained
  Mux3 : Mux  Inputs=2
  Tunable Sigmoid : $bdroot/Tunable Sigmoid  nonlinearity_type=Sigmoid  gain_source=Internal  gain=1  bias=dsyn_pos  slope=msyn_pos
  Tunable Sigmoid1 : $bdroot/Tunable Sigmoid  nonlinearity_type=Sigmoid  gain_source=Internal  gain=1  bias=dsyn_neg  slope=msyn_neg
  VSNK_neg : VariantSink  VariantControlMode=label  LabelModeActiveChoice=Events  ShowConditionOnBlock=on
  VSNK_pos : VariantSink  VariantControlMode=label  LabelModeActiveChoice=Events  ShowConditionOnBlock=on
  VSRC_neg : VariantSource  VariantControlMode=label  LabelModeActiveChoice=Events  ShowConditionOnBlock=on
  VSRC_pos : VariantSource  VariantControlMode=label  LabelModeActiveChoice=Events  ShowConditionOnBlock=on
  base_val : Constant  Value=base_val
  gsyn_neg : Constant  Value=gsyn_neg
  gsyn_pos : Constant  Value=gsyn_pos
  Param : Outport
  wires:
  base_val/1 -> Mux3/2
  Mux3/1 -> Leaky Integration/1
  Leaky Integration/1 -> Param/1
  Ev+/1 -> VSNK_pos/1
  Add22/1 -> Mux3/1
  Isyn_pos/1 -> Add22/1
  Isyn_neg/1 -> Add22/2
  VSNK_pos/1 -> Event to Continuous/1
  Event to Continuous/1 -> VSRC_pos/1
  Tunable Sigmoid/1 -> VSRC_pos/2
  VSNK_pos/2 -> Tunable Sigmoid/1
  VSRC_pos/1 -> Isyn_pos/1
  gsyn_pos/1 -> Isyn_pos/2
  VSRC_neg/1 -> Isyn_neg/1
  gsyn_neg/1 -> Isyn_neg/2
  Event to Continuous1/1 -> VSRC_neg/1
  VSNK_neg/2 -> Tunable Sigmoid1/1
  VSNK_neg/1 -> Event to Continuous1/1
  Tunable Sigmoid1/1 -> VSRC_neg/2
  Ev-/1 -> VSNK_neg/1

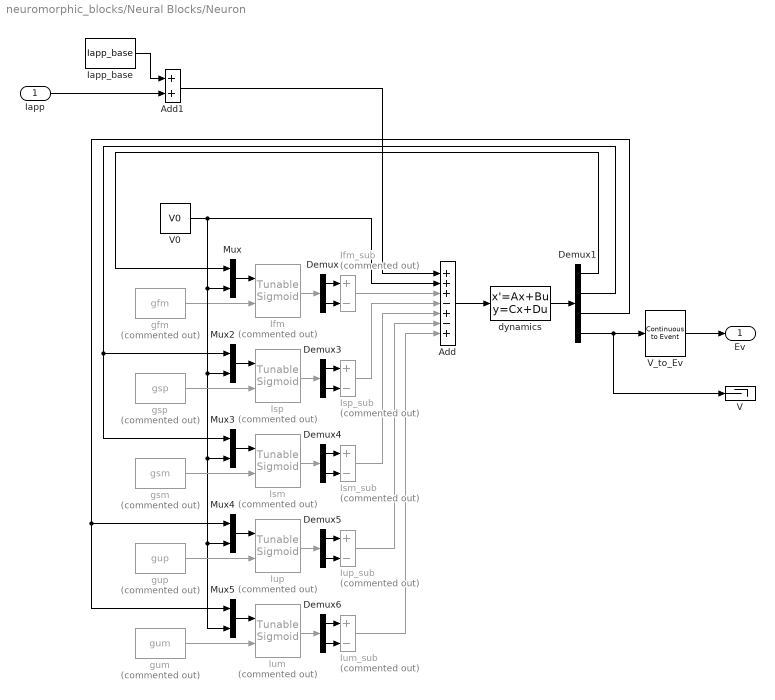
== system neuromorphic_blocks/Neural Blocks/Neuron ==
  Iapp : Inport
  Add : Sum  Inputs=+++-+-+
  Add1 : Sum
  Demux{,3..6} (5 alike) : Demux  Outputs=2
  Demux1 : Demux
  Iapp_base : Constant  Value=Iapp_base
  Ifm : $bdroot/Tunable Sigmoid  Commented=on  nonlinearity_type=Tanh  gain_source=External  gain=0  bias=dfm  slope=mfm
  Ifm_sub : Sum  Commented=on  Inputs=+-
  Ism : $bdroot/Tunable Sigmoid  Commented=on  nonlinearity_type=Tanh  gain_source=External  gain=0  bias=dsm  slope=msm
  Ism_sub : Sum  Commented=on  Inputs=+-
  Isp : $bdroot/Tunable Sigmoid  Commented=on  nonlinearity_type=Tanh  gain_source=External  gain=0  bias=dsp  slope=msp
  Isp_sub : Sum  Commented=on  Inputs=+-
  Ium : $bdroot/Tunable Sigmoid  Commented=on  nonlinearity_type=Tanh  gain_source=External  gain=0  bias=dum  slope=mum
  Ium_sub : Sum  Commented=on  Inputs=+-
  Iup : $bdroot/Tunable Sigmoid  Commented=on  nonlinearity_type=Tanh  gain_source=External  gain=0  bias=dup  slope=mup
  Iup_sub : Sum  Commented=on  Inputs=+-
  Mux{,2..5} (5 alike) : Mux  Inputs=2
  V : Terminator
  V0 : Constant  Value=V0
  V_to_Ev : $bdroot/Events Transmission Blocks/Continuous to Event  thresh=tresh
  dynamics : StateSpace  A=[-1/rel_fast 0 0 1/rel_fast; 0 -1/rel_slow 0 1/rel_slow; 0 0 -1/rel_ultraslow 1/rel_ultraslow; 0 0 0 -1/rel_membrane]/(timescale)  B=[0; 0; 0; 1/rel_membrane]/timescale  C=[1 0 0 0; 0 1 0 0; 0 0 1 0; 0 0 0 1]  D=[0; 0; 0; 0]  InitialCondition=[V0; V0; V0; V0]
  gfm : Constant  Commented=on  Value=gfm
  gsm : Constant  Commented=on  Value=gsm
  gsp : Constant  Commented=on  Value=gsp
  gum : Constant  Commented=on  Value=gum
  gup : Constant  Commented=on  Value=gup
  Ev : Outport
  wires:
  dynamics/1 -> Demux1/1
  Add1/1 -> Add/1
  gfm/1 -> Ifm/2
  Iapp_base/1 -> Add1/1
  Demux1/1 -> Mux/1
  Add/1 -> dynamics/1
  V0/1 -> Mux/2, Mux2/2, Mux5/2, Mux4/2, Mux3/2, Add/2
  Iapp/1 -> Add1/2
  Demux1/3 -> Mux4/1, Mux5/1
  Demux1/4 -> V/1, V_to_Ev/1
  Demux1/2 -> Mux3/1, Mux2/1
  V_to_Ev/1 -> Ev/1
  Mux/1 -> Ifm/1
  Ifm/1 -> Demux/1
  Demux/1 -> Ifm_sub/1
  Demux/2 -> Ifm_sub/2
  Ifm_sub/1 -> Add/3
  Demux3/1 -> Isp_sub/1
  Demux3/2 -> Isp_sub/2
  Mux2/1 -> Isp/1
  Isp/1 -> Demux3/1
  gsp/1 -> Isp/2
  Isp_sub/1 -> Add/4
  Demux4/1 -> Ism_sub/1
  Demux4/2 -> Ism_sub/2
  Mux3/1 -> Ism/1
  Ism/1 -> Demux4/1
  gsm/1 -> Ism/2
  Demux5/1 -> Iup_sub/1
  Demux5/2 -> Iup_sub/2
  Mux4/1 -> Iup/1
  Iup/1 -> Demux5/1
  gup/1 -> Iup/2
  Ism_sub/1 -> Add/5
  Iup_sub/1 -> Add/6
  Ium/1 -> Demux6/1
  Mux5/1 -> Ium/1
  gum/1 -> Ium/2
  Demux6/2 -> Ium_sub/2
  Demux6/1 -> Ium_sub/1
  Ium_sub/1 -> Add/7

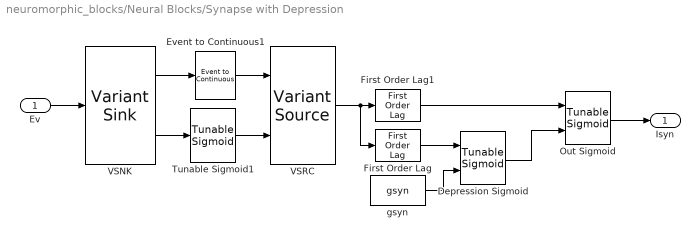
== system neuromorphic_blocks/Neural Blocks/Synapse with Depression ==
  Ev : Inport
  Depression Sigmoid : $bdroot/Tunable Sigmoid  nonlinearity_type=Sigmoid  gain_source=External  gain=0  bias=-dsyn_dep  slope=-msyn_dep
  Event to Continuous1 : $bdroot/Events Transmission Blocks/Event to Continuous  gain=1
  First Order Lag : $bdroot/First Order Lag  gain=1  timescale=timescale  rel_timescale=rel_depression
  First Order Lag1 : $bdroot/First Order Lag  gain=1  timescale=timescale  rel_timescale=rel_facilitation
  Out Sigmoid : $bdroot/Tunable Sigmoid  nonlinearity_type=Sigmoid  gain_source=External  gain=0  bias=dsyn  slope=msyn
  Tunable Sigmoid1 : $bdroot/Tunable Sigmoid  nonlinearity_type=Sigmoid  gain_source=Internal  gain=gsyn_in  bias=dsyn_in  slope=msyn_in
  VSNK : VariantSink  VariantControlMode=label  LabelModeActiveChoice=Events  ShowConditionOnBlock=on
  VSRC : VariantSource  VariantControlMode=label  LabelModeActiveChoice=Events  ShowConditionOnBlock=on
  gsyn : Constant  Value=gsyn
  Isyn : Outport
  wires:
  VSRC/1 -> First Order Lag/1, First Order Lag1/1
  Out Sigmoid/1 -> Isyn/1
  gsyn/1 -> Depression Sigmoid/2
  VSNK/1 -> Event to Continuous1/1
  Event to Continuous1/1 -> VSRC/1
  Tunable Sigmoid1/1 -> VSRC/2
  VSNK/2 -> Tunable Sigmoid1/1
  Ev/1 -> VSNK/1
  Depression Sigmoid/1 -> Out Sigmoid/2
  First Order Lag/1 -> Depression Sigmoid/1
  First Order Lag1/1 -> Out Sigmoid/1

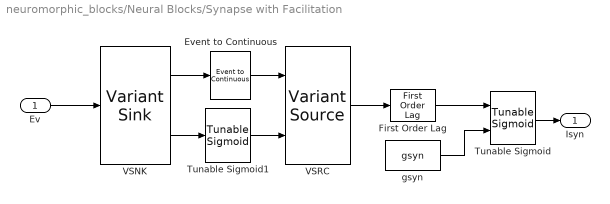
== system neuromorphic_blocks/Neural Blocks/Synapse with Facilitation ==
  Ev : Inport
  Event to Continuous : $bdroot/Events Transmission Blocks/Event to Continuous  gain=1
  First Order Lag : $bdroot/First Order Lag  gain=1  timescale=timescale  rel_timescale=rel_timescale
  Tunable Sigmoid : $bdroot/Tunable Sigmoid  nonlinearity_type=Sigmoid  gain_source=External  gain=0  bias=dsyn  slope=msyn
  Tunable Sigmoid1 : $bdroot/Tunable Sigmoid  nonlinearity_type=Sigmoid  gain_source=Internal  gain=gsyn_in  bias=dsyn_in  slope=msyn_in
  VSNK : VariantSink  VariantControlMode=label  LabelModeActiveChoice=Events  ShowConditionOnBlock=on
  VSRC : VariantSource  VariantControlMode=label  LabelModeActiveChoice=Events  ShowConditionOnBlock=on
  gsyn : Constant  Value=gsyn
  Isyn : Outport
  wires:
  First Order Lag/1 -> Tunable Sigmoid/1
  Tunable Sigmoid/1 -> Isyn/1
  gsyn/1 -> Tunable Sigmoid/2
  Ev/1 -> VSNK/1
  VSNK/2 -> Tunable Sigmoid1/1
  VSNK/1 -> Event to Continuous/1
  Tunable Sigmoid1/1 -> VSRC/2
  Event to Continuous/1 -> VSRC/1
  VSRC/1 -> First Order Lag/1

== system neuromorphic_blocks/Quick Insert/Neural Blocks ==
  Burst Cut Synapse : $bdroot/Neural Blocks/Synapse with Depression  gsyn_source=Internal  gsyn=1  dsyn=2  msyn=10  dsyn_dep=10  msyn_dep=50  timescale=0.004  rel_facilitation=0  rel_depression=100  input=Events  gsyn_in=0  dsyn_in=0  msyn_in=1
  Bursting Neuron : $bdroot/Neural Blocks/Neuron  gfm_source=Internal  gfm=2  gsp_source=Internal  gsp=4  gsm_source=Internal  gsm=2  gup_source=Internal  gup=1.5  gum_source=Internal  gum=0  dfm=0  dsp=0.5  dsm=-0.5  dup=-0.5  dum=-1  mfm=1  msp=1  msm=1  mup=1  mum=1  timescale=0.004  rel_membrane=0.1  rel_fast=0.1  rel_slow=3.1623  rel_ultraslow=100  Iapp_base=-0.2  V0=-1.2  tresh=0  output=Events
  Inhibition Synapse : $bdroot/Neural Blocks/Synapse with Facilitation  gsyn_source=Internal  gsyn=-1  dsyn=4  msyn=10  timescale=0.004  rel_timescale=10  input=Events  gsyn_in=0  dsyn_in=0  msyn_in=1
  Type I Spiking Neuron : $bdroot/Neural Blocks/Neuron  gfm_source=Internal  gfm=2  gsp_source=Internal  gsp=4  gsm_source=Internal  gsm=1  gup_source=Internal  gup=0  gum_source=Internal  gum=0  dfm=0  dsp=0.5  dsm=-0.5  dup=-0.5  dum=-1  mfm=1  msp=1  msm=1  mup=1  mum=1  timescale=0.004  rel_membrane=0.1  rel_fast=0.1  rel_slow=3.1623  rel_ultraslow=100  Iapp_base=-0.12  V0=-1.2  tresh=0  output=Events
  Type II Spiking Neuron1 : $bdroot/Neural Blocks/Neuron  gfm_source=Internal  gfm=2  gsp_source=Internal  gsp=4  gsm_source=Internal  gsm=0  gup_source=Internal  gup=0  gum_source=Internal  gum=0  dfm=0  dsp=0.5  dsm=-0.5  dup=-0.5  dum=-1  mfm=1  msp=1  msm=1  mup=1  mum=1  timescale=0.004  rel_membrane=0.1  rel_fast=0.1  rel_slow=3.1623  rel_ultraslow=100  Iapp_base=0.15  V0=-1.2  tresh=0  output=Events
  Type III Spiking Neuron : $bdroot/Neural Blocks/Neuron  gfm_source=Internal  gfm=2  gsp_source=Internal  gsp=4  gsm_source=Internal  gsm=0  gup_source=Internal  gup=15  gum_source=Internal  gum=0  dfm=0  dsp=0.5  dsm=-0.5  dup=-0.5  dum=-1  mfm=1  msp=1  msm=1  mup=1  mum=1  timescale=0.004  rel_membrane=0.1  rel_fast=0.1  rel_slow=3.1623  rel_ultraslow=100  Iapp_base=0.1  V0=-1.2  tresh=0  output=Events

== system neuromorphic_blocks/Tunable Sigmoid/Sigmoid ==
  x : Inport
  Constant : Constant
  Gain : Gain  Gain=2
  Gain1 : Gain  Gain=0.5
  Sum : Sum  Inputs=|++
  Trigonometric Function : Trigonometry  Operator=tanh
  y : Outport
  wires:
  Gain/1 -> Trigonometric Function/1
  x/1 -> Gain/1
  Trigonometric Function/1 -> Sum/1
  Constant/1 -> Sum/2
  Sum/1 -> Gain1/1
  Gain1/1 -> y/1

== system neuromorphic_blocks/Auxiliary Blocks/Event-Signal Multiplier/VSub ==
  in : Inport
  s : Inport  Port=2
  Events : Subsystem  VariantControl=Events
  Voltage : Subsystem  VariantControl=Voltage
  out+ : Outport
  out- : Outport  Port=2

== system neuromorphic_blocks/Auxiliary Blocks/Event-Signal Selector/VSub ==
  in+ : Inport
  in- : Inport  Port=2
  s : Inport  Port=3
  Events : Subsystem  VariantControl=Events
  Voltage : Subsystem  VariantControl=Voltage
  out : Outport

== system neuromorphic_blocks/Events Transmission Blocks/Event Loss/Generate Random Number on Positive ==
  Trigger : TriggerPort  TriggerType=either  VariantControl=(inherit)  ShowOutputPort=on
  Constant : Constant  Value=0
  Switch : Switch  SaturateOnIntegerOverflow=off  InputSameDT=off
  Uniform Random Number1 : UniformRandomNumber  Minimum=0  Seed=seed_mem
  Out1 : Outport
  wires:
  Constant/1 -> Switch/3
  Trigger/1 -> Switch/2
  Uniform Random Number1/1 -> Switch/1
  Switch/1 -> Out1/1

== system neuromorphic_blocks/Events Transmission Blocks/Event to Fixed Width Pulse/Triggered Subsystem ==
  In1 : Inport
  Trigger : TriggerPort  VariantControl=(inherit)  InitialTriggerSignalState=zero
  Out1 : Outport  InitialOutput=-pulse_width
  wires:
  In1/1 -> Out1/1
